simulink model "generate_timeseries"  (R2016b)
settings: Solver=FixedStepDiscrete  StartTime=0.0  StopTime=10  FixedStep=0.01  RelTol=1e-3
InitFcn:
  | run('enum_definition.m')
libraries: simulink x1
settings Model: Creator=T8100AV  LastModifiedBy=T8100AV
settings DataIOCC: SaveOutput=off  StreamToWorkspace=on  SaveTime=off

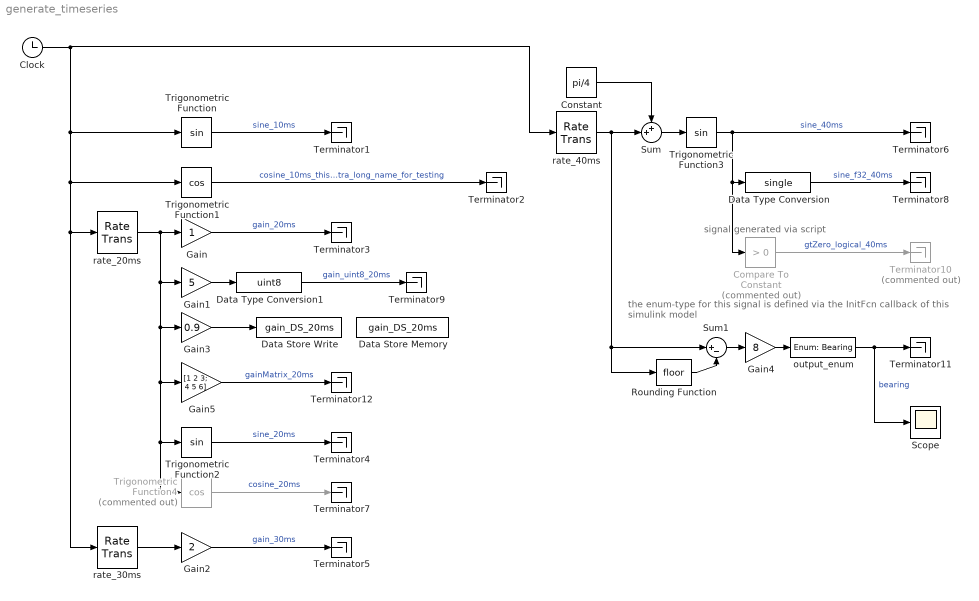
== system generate_timeseries ==
  note: the enum-type for this signal is defined via the InitFcn
      | callback of this simulink model
  note: signal generated via script
  Clock : Clock
  Compare To Constant : simulink/Logic and Bit Operations/Compare To Constant  Commented=on  relop=>  const=0  OutDataTypeStr=boolean
  Constant : Constant  Value=pi/4
  Data Store Memory : DataStoreMemory  DataStoreName=gain_DS_20ms  ReadBeforeWriteMsg=warning  WriteAfterWriteMsg=warning  WriteAfterReadMsg=warning  ShowAdditionalParam=off
  Data Store Write : DataStoreWrite  DataStoreName=gain_DS_20ms
  Data Type Conversion : DataTypeConversion  OutDataTypeStr=single
  Data Type Conversion1 : DataTypeConversion  OutDataTypeStr=uint8
  Gain : Gain
  Gain1 : Gain  Gain=5  OutDataTypeStr=double
  Gain2 : Gain  Gain=2
  Gain3 : Gain  Gain=0.9
  Gain4 : Gain  Gain=8  OutDataTypeStr=int32
  Gain5 : Gain  Gain=[1 2 3; 4 5 6]
  Rounding Function : Rounding
  Scope : Scope
  Sum : Sum  Inputs=++|
  Sum1 : Sum  Inputs=|+-
  Terminator{1..9,11..12} (11 alike) : Terminator
  Terminator10 : Terminator  Commented=on
  Trigonometric Function : Trigonometry
  Trigonometric Function1 : Trigonometry  Operator=cos
  Trigonometric Function2 : Trigonometry
  Trigonometric Function3 : Trigonometry
  Trigonometric Function4 : Trigonometry  Commented=on  Operator=cos
  output_enum : DataTypeConversion  OutDataTypeStr=Enum: Bearing
  rate_20ms : RateTransition  OutPortSampleTime=0.02
  rate_30ms : RateTransition  OutPortSampleTime=0.03
  rate_40ms : RateTransition  OutPortSampleTime=0.04
  wires:
  Trigonometric Function/1 -> Terminator1/1  "sine_10ms"
  Trigonometric Function1/1 -> Terminator2/1  "cosine_10ms_this_is_an_extra_long_name_for_testing"
  Gain/1 -> Terminator3/1  "gain_20ms"
  Trigonometric Function2/1 -> Terminator4/1  "sine_20ms"
  rate_30ms/1 -> Gain2/1
  Gain2/1 -> Terminator5/1  "gain_30ms"
  Trigonometric Function3/1 -> Compare To Constant/1, Data Type Conversion/1, Terminator6/1  "sine_40ms"
  Sum/1 -> Trigonometric Function3/1
  Trigonometric Function4/1 -> Terminator7/1  "cosine_20ms"
  Data Type Conversion/1 -> Terminator8/1  "sine_f32_40ms"
  Gain1/1 -> Data Type Conversion1/1
  Data Type Conversion1/1 -> Terminator9/1  "gain_uint8_20ms"
  Compare To Constant/1 -> Terminator10/1  "gtZero_logical_40ms"
  Gain3/1 -> Data Store Write/1
  Clock/1 -> rate_30ms/1, rate_20ms/1, Trigonometric Function1/1, Trigonometric Function/1, rate_40ms/1
  rate_40ms/1 -> Sum1/1, Rounding Function/1, Sum/2
  Rounding Function/1 -> Sum1/2
  Sum1/1 -> Gain4/1
  Gain4/1 -> output_enum/1
  output_enum/1 -> Scope/1, Terminator11/1  "bearing"
  Constant/1 -> Sum/1
  rate_20ms/1 -> Gain3/1, Gain5/1, Trigonometric Function4/1, Trigonometric Function2/1, Gain1/1, Gain/1
  Gain5/1 -> Terminator12/1  "gainMatrix_20ms"
